simulink subsystem "TOAD_Controller_2"  (R2025b)
settings: Solver=VariableStepAuto  StartTime=0.0  StopTime=10.0  RelTol=1e-3
undefined symbols (not defined in the file or in its folder): constantsTOAD, DiscIntNeverNeededParam, dt_SIM, u0
settings Model: Creator=pplat  LastModifiedBy=pplat

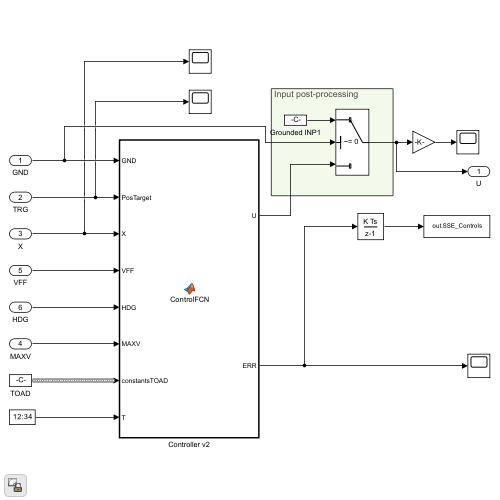
[thumbnail: Simulink's stored preview of the top-level diagram]
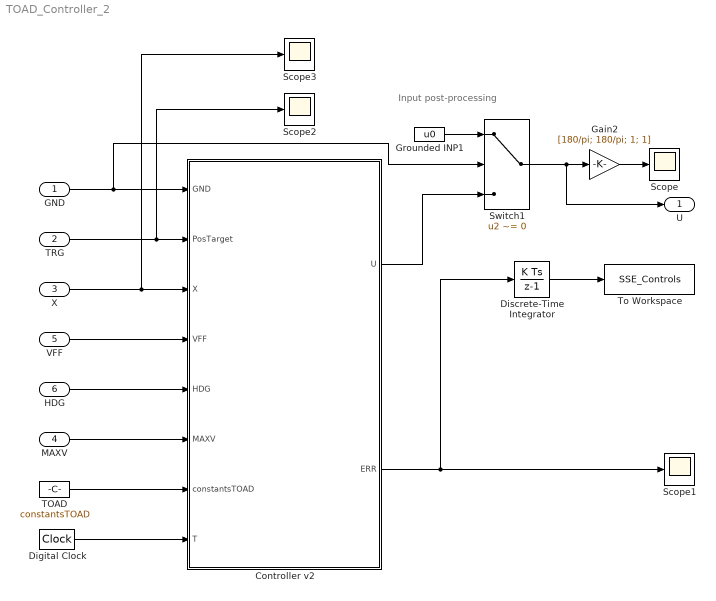
== system TOAD_Controller_2 ==
  note: Input post-processing
  GND : Inport
  TRG : Inport  Port=2  PortDimensions=[3, 1]
  X : Inport  Port=3  PortDimensions=[15, 1]
  MAXV : Inport  Port=4  PortDimensions=[3, 1]
  VFF : Inport  Port=5  PortDimensions=[3,1]
  HDG : Inport  Port=6
  Controller v2 : MATLAB Function  TreatAsAtomicUnit=on
  Digital Clock : DigitalClock  SampleTime=dt_SIM
  Discrete-Time Integrator : DiscreteIntegrator  InitialCondition=zeros(9,1)  SampleTime=-1  ICPrevOutput=DiscIntNeverNeededParam  ICPrevScaledInput=DiscIntNeverNeededParam
  Gain2 : Gain  Gain=[180/pi; 180/pi; 1; 1]
  Grounded INP1 : Constant  Value=u0
  Scope{,1..3} (4 alike) : Scope
      Scope settings: ActiveDisplayYMinimum=-11.801195540279929  ActiveDisplayYMaximum=6.2107598625193638  DataLoggingVariableName=ScopeData8
      Scope1 settings: ActiveDisplayYMinimum=-2.0506088304624521  ActiveDisplayYMaximum=3.7155232700223415  DataLoggingVariableName=ScopeData13
      Scope2 settings: ActiveDisplayYMinimum=-1  ActiveDisplayYMaximum=1  DataLoggingVariableName=ScopeData18
      Scope3 settings: ActiveDisplayYMinimum=-0.53566092037557744  ActiveDisplayYMaximum=3.4212061004598149  DataLoggingVariableName=ScopeData19
  Switch1 : Switch  Criteria=u2 ~= 0  SaturateOnIntegerOverflow=off  InputSameDT=off
  TOAD : Constant  Value=constantsTOAD  OutDataTypeStr=Bus: slBus1
  To Workspace : ToWorkspace  VariableName=SSE_Controls  SampleTime=-1
      settings: MaxDataPoints=1
  U : Outport
  wires:
  Gain2/1 -> Scope/1
  X/1 -> Scope3/1, Controller v2/3(X)
  HDG/1 -> Controller v2/5(HDG)
  VFF/1 -> Controller v2/4(VFF)
  GND/1 -> Switch1/2, Controller v2/1(GND)
  Digital Clock/1 -> Controller v2/8(T)
  Controller v2/1(U) -> Switch1/3
  Switch1/1 -> Gain2/1, U/1
  Grounded INP1/1 -> Switch1/1
  TRG/1 -> Scope2/1, Controller v2/2(PosTarget)
  TOAD/1 -> Controller v2/7(constantsTOAD)
  Controller v2/2(ERR) -> Scope1/1, Discrete-Time Integrator/1
  Discrete-Time Integrator/1 -> To Workspace/1
  MAXV/1 -> Controller v2/6(MAXV)

== matlab function TOAD_Controller_2/Controller v2 ==
  data: GND input; PosTarget input; X input; VFF input; HDG input; MAXV input; constantsTOAD input; U output; T input; ERR output
function [U, ERR] = ControlFCN(GND, PosTarget, X, VFF, HDG, MAXV,constantsTOAD,  T)

    [U, ERR] = TOAD_Control_FCN(PosTarget, X, constantsTOAD,  T, MAXV, VFF, HDG, GND);
